simulink model "SUS_ST_GUI"  (R2014a)
settings: Solver=ode3  StartTime=0.0  StopTime=T  FixedStep=0.1  RelTol=1e-3
values from neighbouring files (symbols this model uses):
  CA = str2double(get(handles.CA,'string'))    [SUS_ST_0326.m]    (also in SUS_ST_GUI_0326.m)
  IN = str2double(get(handles.IN,'string'))    [SUS_ST_0326.m]    (also in SUS_ST_GUI_0326.m)
  LT = str2double(get(handles.LT,'string'))    [SUS_ST_GUI_0326.m]
  N = 1    [SUS_ST_0326.m]
  SR = str2double(get(handles.SR,'string'))    [SUS_ST_0326.m]    (also in SUS_ST_GUI_0326.m)
  ST = str2double(get(handles.ST,'string'))    [SUS_ST_GUI_0326.m]
  ST_S = str2double(get(handles.ST_S,'string'))    [SUS_ST_GUI_0326.m]
  T = 10    [SUS_ST_GUI_0326.m]
  T5 = str2double(get(handles.T5,'string'))    [SUS_ST_0326.m]    (also in SUS_ST_GUI_0326.m)
  T6 = str2double(get(handles.T6,'string'))    [SUS_ST_0326.m]    (also in SUS_ST_GUI_0326.m)
  X11 = (Z11-H/sind(CA)-b2_3)/k2_3    [SUS_ST_GUI_0326.m]
  X12 = (Z12-bb2_3)/k2_3    [SUS_ST_GUI_0326.m]
  X13 = X12-X12_3    [SUS_ST_GUI_0326.m]
  X14 = X9+X14_1    [SUS_ST_GUI_0326.m]
  X15 = X9+X15_1    [SUS_ST_GUI_0326.m]
  X16 = X9+X16_2    [SUS_ST_GUI_0326.m]
  X2 = -abs(Z3)*tand(CA)    [SUS_ST_GUI_0326.m]
  x2 = 0    [SUS_ST_GUI_0326.m]
  X3 = abs(Z2)*tand(CA)    [SUS_ST_GUI_0326.m]
  x3 = 0    [SUS_ST_GUI_0326.m]
  x4 = str2double(get(handles.x4,'string'))    [SUS_ST_0326.m]    (also in SUS_ST_GUI_0326.m)
  X5 = X4-a1*cosd(T5)    [SUS_ST_GUI_0326.m]
  x5 = 0    [SUS_ST_GUI_0326.m]
  X6 = X4+b1*cosd(T5)    [SUS_ST_GUI_0326.m]
  x6 = str2double(get(handles.x6,'string'))    [SUS_ST_0326.m]    (also in SUS_ST_GUI_0326.m)
  X7 = X1-a2*cosd(T6)    [SUS_ST_GUI_0326.m]
  x7 = x4-e7    [SUS_ST_GUI_0326.m]
  X8 = X1+b2*cosd(T6)    [SUS_ST_GUI_0326.m]
  x8 = x9-l8*sind(t8)    [SUS_ST_GUI_0326.m]
  X9 = str2double(get(handles.X9,'string'))    [SUS_ST_0326.m]    (also in SUS_ST_GUI_0326.m)
  x9 = str2double(get(handles.x9,'string'))    [SUS_ST_0326.m]    (also in SUS_ST_GUI_0326.m)
  XC1 = (X7+X2+X8)/3    [SUS_ST_GUI_0326.m]
  xc1 = (x3+x4+x5)/3    [SUS_ST_GUI_0326.m]
  XC2 = (X3+X2)/2    [SUS_ST_GUI_0326.m]
  XC3 = (X5+X3+X6)/3    [SUS_ST_GUI_0326.m]
  Y11 = M/2    [SUS_ST_GUI_0326.m]
  Y12 = (B11_12-BB2_3)/(K2_3-K11_12)    [SUS_ST_GUI_0326.m]
  Y13 = Y12-Y12_3    [SUS_ST_GUI_0326.m]
  Y14 = Y9+Y14_1    [SUS_ST_GUI_0326.m]
  Y15 = Y9+Y15_1    [SUS_ST_GUI_0326.m]
  Y16 = Y9+Y16_2    [SUS_ST_GUI_0326.m]
  Y2 = (Z2-Z9)/K2_3+Y9-SR    [SUS_ST_GUI_0326.m]
  y2 = Y1+l2*cosd(t2+T2)    [SUS_ST_GUI_0326.m]
  Y3 = (Z3-Z9)/K2_3+Y9-SR    [SUS_ST_GUI_0326.m]
  y3 = y4+l4*cosd(t4)    [SUS_ST_GUI_0326.m]
  y4 = str2double(get(handles.y4,'string'))    [SUS_ST_0326.m]    (also in SUS_ST_GUI_0326.m)
  Y5 = Y4    [SUS_ST_GUI_0326.m]
  y5 = y4+l5*cosd(t5)    [SUS_ST_GUI_0326.m]
  Y6 = Y4    [SUS_ST_GUI_0326.m]
  y6 = str2double(get(handles.y6,'string'))    [SUS_ST_0326.m]    (also in SUS_ST_GUI_0326.m)
  Y7 = Y1    [SUS_ST_GUI_0326.m]
  y7 = y4+l7*cosd(t7)    [SUS_ST_GUI_0326.m]
  Y8 = Y1    [SUS_ST_GUI_0326.m]
  y8 = y9+l8*cosd(t8)    [SUS_ST_GUI_0326.m]
  Y9 = str2double(get(handles.Y9,'string'))    [SUS_ST_0326.m]    (also in SUS_ST_GUI_0326.m)
  y9 = str2double(get(handles.y9,'string'))    [SUS_ST_0326.m]    (also in SUS_ST_GUI_0326.m)
  YC1 = (Y7+Y2+Y8)/3    [SUS_ST_GUI_0326.m]
  yc1 = (y3+y4+y5)/3    [SUS_ST_GUI_0326.m]
  YC2 = (Y3+Y2)/2    [SUS_ST_GUI_0326.m]
  YC3 = (Y5+Y3+Y6)/3    [SUS_ST_GUI_0326.m]
  Z11 = str2double(get(handles.Z11,'string'))    [SUS_ST_0326.m]    (also in SUS_ST_GUI_0326.m)
  Z12 = str2double(get(handles.Z12,'string'))    [SUS_ST_0326.m]    (also in SUS_ST_GUI_0326.m = K11_12*Y12+B11_12)
  Z13 = Z12-Z12_3    [SUS_ST_GUI_0326.m]
  Z14 = Z9+Z14_1    [SUS_ST_GUI_0326.m]
  Z15 = Z9+Z15_1    [SUS_ST_GUI_0326.m]
  Z16 = Z9+Z16_2    [SUS_ST_GUI_0326.m]
  Z2 = str2double(get(handles.Z2,'string'))    [SUS_ST_0326.m]    (also in SUS_ST_GUI_0326.m)
  z2 = Z1+l2*sind(t2+T2)    [SUS_ST_GUI_0326.m]
  Z3 = str2double(get(handles.Z3,'string'))    [SUS_ST_0326.m]    (also in SUS_ST_GUI_0326.m)
  z3 = z4+l4*sind(t4)    [SUS_ST_GUI_0326.m]
  z4 = str2double(get(handles.z4,'string'))    [SUS_ST_0326.m]    (also in SUS_ST_GUI_0326.m)
  Z5 = Z4-a1*sind(T5)    [SUS_ST_GUI_0326.m]
  z5 = z4+l5*sind(t5)    [SUS_ST_GUI_0326.m]
  Z6 = Z4+b1*sind(T5)    [SUS_ST_GUI_0326.m]
  z6 = str2double(get(handles.z6,'string'))    [SUS_ST_0326.m]    (also in SUS_ST_GUI_0326.m)
  Z7 = Z1-a2*sind(T6)    [SUS_ST_GUI_0326.m]
  z7 = z4+l7*sind(t7)    [SUS_ST_GUI_0326.m]
  Z8 = Z1+b2*sind(T6)    [SUS_ST_GUI_0326.m]
  z8 = z9    [SUS_ST_GUI_0326.m]
  Z9 = str2double(get(handles.Z9,'string'))    [SUS_ST_0326.m]    (also in SUS_ST_GUI_0326.m)
  z9 = str2double(get(handles.z9,'string'))    [SUS_ST_0326.m]    (also in SUS_ST_GUI_0326.m)
  ZC1 = (Z7+Z2+Z8)/3    [SUS_ST_GUI_0326.m]
  zc1 = (z3+z4+z5)/3    [SUS_ST_GUI_0326.m]
  ZC2 = (Z3+Z2)/2    [SUS_ST_GUI_0326.m]
  ZC3 = (Z5+Z3+Z6)/3    [SUS_ST_GUI_0326.m]
libraries: mblibv1 x79, simulink x3
(part 1 of 2)
settings Model: Creator=Administrator  LastModifiedBy=ZBingF
settings DebuggingCC: UnderspecifiedInitializationDetection=Classic  StateNameClashWarn=warning
settings SimMechanicsCC: VisDuringSimulation=on

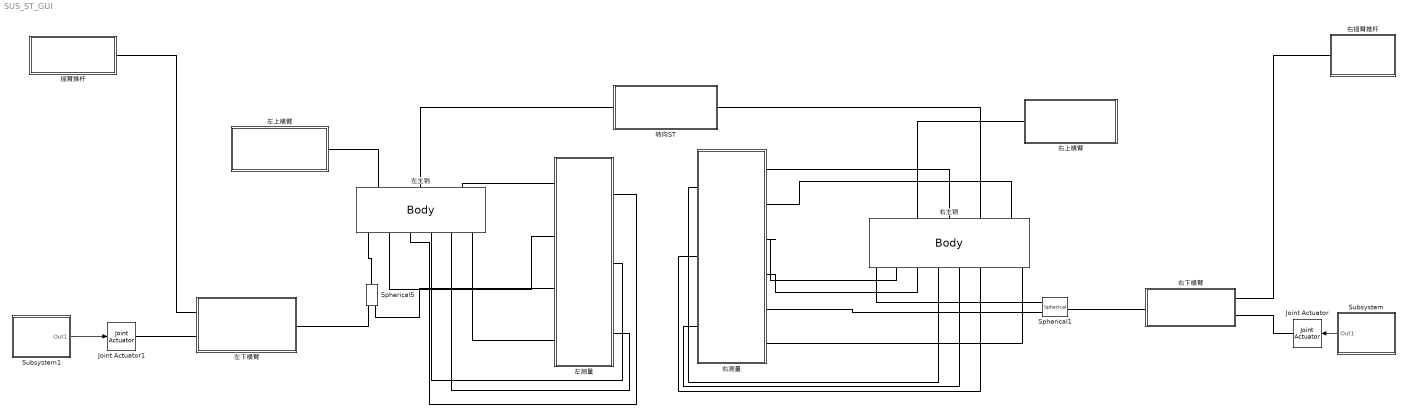
== system SUS_ST_GUI ==
  Joint Actuator : mblibv1/Sensors &  Actuators/Joint Actuator  UpdateFromCAD=off  PhysicalDomain=Mechanical  PortType=blob  ActuationStyle=Motion  AngleUnits=deg  ArcVelocityUnits=deg/s  ArcAccelerationUnits=deg/s^2  CoordPositionUnits=m  VelocityUnits=m/s  AccelerationUnits=m/s^2  ForceUnits=N  TorqueUnits=N*m  ActiveIO=on  Width=3  DialogClass=MechanicalActuatorBlock  Primitive=R1  ReferenceFrame=Absolute (World)
  Joint Actuator1 : mblibv1/Sensors &  Actuators/Joint Actuator  UpdateFromCAD=off  PhysicalDomain=Mechanical  PortType=blob  ActuationStyle=Motion  AngleUnits=deg  ArcVelocityUnits=deg/s  ArcAccelerationUnits=deg/s^2  CoordPositionUnits=m  VelocityUnits=m/s  AccelerationUnits=m/s^2  ForceUnits=N  TorqueUnits=N*m  ActiveIO=on  Width=3  DialogClass=MechanicalActuatorBlock  Primitive=R1  ReferenceFrame=Absolute (World)
  Spherical1 : mblibv1/Joints/Spherical  LConnTagsString=__newl0|SA1  RConnTagsString=__newr0  UpdateFromCAD=off  NumSAPorts=1  CutJoint=off  MarkAsCut=off  Primitives=spherical  PrimitiveProps=S$World$[0 0 0]$spherical  DialogClass=JointBlock  SAxis=[0 0 0]
  Spherical5 : mblibv1/Joints/Spherical  LConnTagsString=__newl0|SA1  RConnTagsString=__newr0  UpdateFromCAD=off  NumSAPorts=1  CutJoint=off  MarkAsCut=off  Primitives=spherical  PrimitiveProps=S$World$[0 0 0]$spherical  DialogClass=JointBlock  SAxis=[0 0 0]
  Subsystem : Subsystem
  Subsystem1 : Subsystem
  右上横臂 : Subsystem
  右下横臂 : Subsystem
  右主销 : mblibv1/Bodies/Body  LConnTagsString=CG|CS1|CS4|CS6|CS7  RConnTagsString=CS2|CS5|CS3|CS10|CS12|CS11|CS9|CS8  UpdateFromCAD=off  DialogClass=MechanicalBodyBlock  Mass=1  MassUnits=kg  InertiaUnits=kg*m^2  Inertia=eye(3)  Shape=Cylinder  ShapeDims=[1 1]  ShapeUnits=m  ShapeUse=false  Density=1  DensityUnits=kg/m^3  DensityUse=false  GraphicsMode=MACHINE_DEFAULT  BodyColorSelMode=MACHINE_DEFAULT  BodyColor=[1 0 0]  AttachedToCS=CG  CG=Left$CG$[XC2 YC2 ZC2]$WORLD$WORLD$mm$[0 0 0]$Euler X-Y-Z$deg$WORLD$true$none  WorkingFrames=Left$CS1$[X3 Y3 Z3]$World$World$mm$[0 0 0]$Euler X-Y-Z$deg$WORLD$true$none#Left$CS4$[X3 Y3 Z3]$World$World$mm$[0 0 0]$Euler X-Y-Z$deg$WORLD$true$none#Right$CS2$[X2 Y2 Z2]$World$World$mm$[IN CA 0]$Euler X-Y-Z$deg$WORLD$true$none#Right$CS5$[X2 Y2 Z2]$World$World$mm$[0 0 0]$Euler X-Y-Z$deg$WORLD$true$none#Right$CS3$[X9 Y9 Z9]$World$World$mm$[0 0 0]$Euler X-Y-Z$deg$WORLD$true$none#Right$CS10$[X14 Y14 Z14]$World$World$mm$[0 0 0]$Euler X-Y-Z$deg$WORLD$true$none#Right$CS12$[X16 Y16 Z16]$World$World$mm$[0 0 0]$Euler X-Y-Z$deg$WORLD$true$none#Right$CS11$[X15 Y15 Z15]$World$World$mm$[0 0 0]$Euler X-Y-Z$deg$WORLD$true$none#Right$CS9$[X9 Y9-SR Z9]$World$World$mm$[IN CA 0]$Euler X-Y-Z$deg$WORLD$true$none#Left$CS6$[X12 Y12 Z12]$World$World$mm$[0 0 0]$Euler X-Y-Z$deg$WORLD$true$none#Left$CS7$[X12 Y12 Z12]$World$World$mm$[0 0 0]$Euler X-Y-Z$deg$WORLD$true$none#Right$CS8$[X13 Y13 Z13]$World$World$mm$[0 0 0]$Euler X-Y-Z$deg$WORLD$true$none  CGPos=[XC2 YC2 ZC2]  CGRot=[0 0 0]  CS0Pos=[]  CS0Rot=[]  CS1Pos=[X3 Y3 Z3]  CS1Rot=[0 0 0]  CS2Pos=[X2 Y2 Z2]  CS2Rot=[IN CA 0]  CS3Pos=[X9 Y9 Z9]  CS3Rot=[0 0 0]  CS4Pos=[X3 Y3 Z3]  CS4Rot=[0 0 0]  CS5Pos=[X2 Y2 Z2]  CS5Rot=[0 0 0]  CS6Pos=[X12 Y12 Z12]  CS6Rot=[0 0 0]  CS7Pos=[X12 Y12 Z12]  CS7Rot=[0 0 0]  CS8Pos=[X13 Y13 Z13]  CS8Rot=[0 0 0]  CS9Pos=[X9 Y9-SR Z9]  CS9Rot=[IN CA 0]  CS10Pos=[X14 Y14 Z14]  CS10Rot=[0 0 0]  CS11Pos=[X15 Y15 Z15]  CS11Rot=[0 0 0]  CS12Pos=[X16 Y16 Z16]  CS12Rot=[0 0 0]  CS13Pos=[]  CS13Rot=[]  CS14Pos=[]  CS14Rot=[]  CS15Pos=[]  CS15Rot=[]  CS16Pos=[]  CS16Rot=[]  CS17Pos=[]  CS17Rot=[]  CS18Pos=[]  CS18Rot=[]  CS19Pos=[]  CS19Rot=[]  CS20Pos=[]  CS20Rot=[]
  右摇臂推杆 : Subsystem
  右测量 : Subsystem
  左上横臂 : Subsystem
  左下横臂 : Subsystem
  左主销 : mblibv1/Bodies/Body  LConnTagsString=CS1|CS6|CS7  RConnTagsString=CS2|CS3|CS9|CS10|CS11|CS8  UpdateFromCAD=off  DialogClass=MechanicalBodyBlock  Mass=1  MassUnits=kg  InertiaUnits=kg*m^2  Inertia=eye(3)  Shape=Cylinder  ShapeDims=[1 1]  ShapeUnits=m  ShapeUse=false  Density=1  DensityUnits=kg/m^3  DensityUse=false  GraphicsMode=MACHINE_DEFAULT  BodyColorSelMode=MACHINE_DEFAULT  BodyColor=[1 0 0]  AttachedToCS=CG  CG=Left$CG$[XC2 -YC2 ZC2]$WORLD$WORLD$mm$[0 0 0]$Euler X-Y-Z$deg$WORLD$false$none  WorkingFrames=Left$CS1$[X3 -Y3 Z3]$World$World$mm$[0 0 0]$Euler X-Y-Z$deg$WORLD$true$none#Left$CS4$[X3 -Y3 Z3]$World$World$mm$[0 0 0]$Euler X-Y-Z$deg$WORLD$false$none#Right$CS2$[X2 -Y2 Z2]$World$World$mm$[-IN CA 0]$Euler X-Y-Z$deg$WORLD$true$none#Right$CS5$[X2 -Y2 Z2]$World$World$mm$[0 0 0]$Euler X-Y-Z$deg$WORLD$false$none#Right$CS3$[X9 -Y9 Z9]$World$World$mm$[0 0 0]$Euler X-Y-Z$deg$WORLD$true$none#Right$CS9$[X14 -Y14 Z14]$World$World$mm$[0 0 0]$Euler X-Y-Z$deg$WORLD$true$none#Right$CS10$[X15 -Y15 Z15]$World$World$mm$[0 0 0]$Euler X-Y-Z$deg$WORLD$true$none#Right$CS11$[X16 -Y16 Z16]$World$World$mm$[0 0 0]$Euler X-Y-Z$deg$WORLD$true$none#Right$CS8$[X13 -Y13 Z13]$World$World$mm$[0 0 0]$Euler X-Y-Z$deg$WORLD$true$none#Left$CS6$[X12 -Y12 Z12]$World$World$mm$[0 0 0]$Euler X-Y-Z$deg$WORLD$true$none#Left$CS7$[X12 -Y12 Z12]$World$World$mm$[0 0 0]$Euler X-Y-Z$deg$WORLD$true$none  CGPos=[XC2 -YC2 ZC2]  CGRot=[0 0 0]  CS0Pos=[]  CS0Rot=[]  CS1Pos=[X3 -Y3 Z3]  CS1Rot=[0 0 0]  CS2Pos=[X2 -Y2 Z2]  CS2Rot=[-IN CA 0]  CS3Pos=[X9 -Y9 Z9]  CS3Rot=[0 0 0]  CS4Pos=[X3 -Y3 Z3]  CS4Rot=[0 0 0]  CS5Pos=[X2 -Y2 Z2]  CS5Rot=[0 0 0]  CS6Pos=[X12 -Y12 Z12]  CS6Rot=[0 0 0]  CS7Pos=[X12 -Y12 Z12]  CS7Rot=[0 0 0]  CS8Pos=[X13 -Y13 Z13]  CS8Rot=[0 0 0]  CS9Pos=[X14 -Y14 Z14]  CS9Rot=[0 0 0]  CS10Pos=[X15 -Y15 Z15]  CS10Rot=[0 0 0]  CS11Pos=[X16 -Y16 Z16]  CS11Rot=[0 0 0]  CS12Pos=[]  CS12Rot=[]  CS13Pos=[]  CS13Rot=[]  CS14Pos=[]  CS14Rot=[]  CS15Pos=[]  CS15Rot=[]  CS16Pos=[]  CS16Rot=[]  CS17Pos=[]  CS17Rot=[]  CS18Pos=[]  CS18Rot=[]  CS19Pos=[]  CS19Rot=[]  CS20Pos=[]  CS20Rot=[]
  左测量 : Subsystem
  摇臂推杆 : Subsystem
  转向ST : Subsystem
  wires:
  Subsystem/1(Out1) -> Joint Actuator/1
  Subsystem1/1(Out1) -> Joint Actuator1/1
  connections:
  右主销/RConn1 -- Spherical1/LConn1
  Spherical5/RConn1 -- 左主销/RConn1
  左主销/LConn2 -- 转向ST/LConn1
  右主销/LConn4 -- 转向ST/RConn1
  左上横臂/LConn1 -- 左主销/LConn1
  左下横臂/LConn1 -- 摇臂推杆/RConn1
  左下横臂/RConn1 -- Spherical5/LConn1
  Joint Actuator1/RConn1 -- 左下横臂/LConn2
  右主销/LConn2 -- 右上横臂/LConn1
  右摇臂推杆/RConn1 -- 右下横臂/LConn1
  右下横臂/RConn1 -- Spherical1/RConn1
  Joint Actuator/RConn1 -- 右下横臂/LConn2
  右测量/RConn1 -- 右主销/LConn3
  右测量/RConn2 -- 右主销/LConn5
  右测量/RConn3 -- 右主销/RConn2
  右测量/RConn4 -- 右主销/RConn3
  右测量/RConn5 -- Spherical1/LConn2
  左测量/LConn1 -- 左主销/LConn3
  左主销/RConn2 -- 左测量/LConn2
  左测量/LConn3 -- Spherical5/LConn2
  左测量/LConn4 -- 左主销/RConn6
  右测量/RConn6 -- 右主销/RConn8
  右测量/LConn1 -- 右主销/RConn4
  右测量/LConn2 -- 右主销/RConn6
  左测量/RConn1 -- 左主销/RConn3
  左测量/RConn2 -- 左主销/RConn4
  右测量/LConn3 -- 右主销/RConn5
  左主销/RConn5 -- 左测量/RConn3

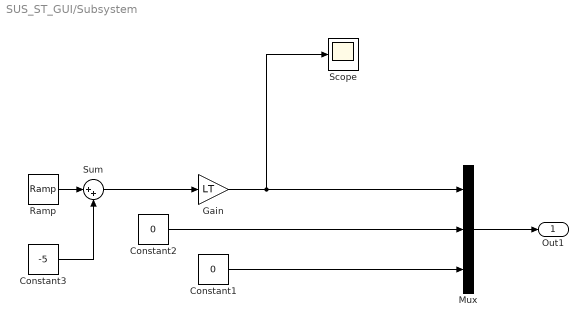
== system SUS_ST_GUI/Subsystem ==
  Constant1 : Constant  Value=0
  Constant2 : Constant  Value=0
  Constant3 : Constant  Value=-5
  Gain : Gain  Gain=LT
  Mux : Mux  Inputs=3
  Ramp : simulink/Sources/Ramp  slope=1  start=0  X0=0
  Scope : Scope
      settings: SaveName=ScopeData3
  Sum : Sum  Inputs=|++
  Out1 : Outport
  wires:
  Mux/1 -> Out1/1
  Gain/1 -> Scope/1, Mux/1
  Constant1/1 -> Mux/3
  Constant2/1 -> Mux/2
  Ramp/1 -> Sum/1
  Constant3/1 -> Sum/2
  Sum/1 -> Gain/1

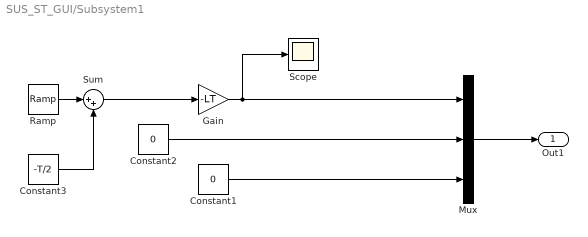
== system SUS_ST_GUI/Subsystem1 ==
  Constant1 : Constant  Value=0
  Constant2 : Constant  Value=0
  Constant3 : Constant  Value=-T/2
  Gain : Gain  Gain=-LT
  Mux : Mux  Inputs=3
  Ramp : simulink/Sources/Ramp  slope=1  start=0  X0=0
  Scope : Scope
      settings: SaveName=ScopeData2
  Sum : Sum  Inputs=|++
  Out1 : Outport
  wires:
  Mux/1 -> Out1/1
  Gain/1 -> Scope/1, Mux/1
  Constant1/1 -> Mux/3
  Constant2/1 -> Mux/2
  Ramp/1 -> Sum/1
  Constant3/1 -> Sum/2
  Sum/1 -> Gain/1

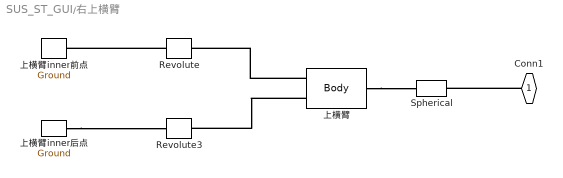
== system SUS_ST_GUI/右上横臂 ==
  Revolute : mblibv1/Joints/Revolute  LConnTagsString=__newl0  RConnTagsString=__newr0  UpdateFromCAD=off  NumSAPorts=0  CutJoint=off  MarkAsCut=off  Primitives=prismatic  PrimitiveProps=R1$World$[cosd(T5) 0 sind(T5)]$revolute  DialogClass=JointBlock  R1Axis=[cosd(T5) 0 sind(T5)]
  Revolute3 : mblibv1/Joints/Revolute  LConnTagsString=__newl0  RConnTagsString=__newr0  UpdateFromCAD=off  NumSAPorts=0  CutJoint=off  MarkAsCut=off  Primitives=prismatic  PrimitiveProps=R1$World$[cosd(T5) 0 sind(T5)]$revolute  DialogClass=JointBlock  R1Axis=[cosd(T5) 0 sind(T5)]
  Spherical : mblibv1/Joints/Spherical  LConnTagsString=__newl0  RConnTagsString=__newr0  UpdateFromCAD=off  NumSAPorts=0  CutJoint=off  MarkAsCut=off  Primitives=spherical  PrimitiveProps=S$World$[0 0 0]$spherical  DialogClass=JointBlock  SAxis=[0 0 0]
  上横臂 : mblibv1/Bodies/Body  LConnTagsString=CS1|CS3  RConnTagsString=CS2  UpdateFromCAD=off  DialogClass=MechanicalBodyBlock  Mass=1  MassUnits=kg  InertiaUnits=kg*m^2  Inertia=eye(3)  Shape=Cylinder  ShapeDims=[1 1]  ShapeUnits=m  ShapeUse=false  Density=1  DensityUnits=kg/m^3  DensityUse=false  GraphicsMode=MACHINE_DEFAULT  BodyColorSelMode=MACHINE_DEFAULT  BodyColor=[1 0 0]  AttachedToCS=CG  CG=Left$CG$[XC3 YC3 ZC3]$WORLD$WORLD$mm$[0 0 0]$Euler X-Y-Z$deg$WORLD$false$none  WorkingFrames=Left$CS1$[X5 Y5 Z5]$World$World$mm$[0 0 0]$Euler X-Y-Z$deg$WORLD$true$none#Right$CS2$[X3 Y3 Z3]$World$World$mm$[0 0 0]$Euler X-Y-Z$deg$WORLD$true$none#Left$CS3$[X6 Y6 Z6]$World$World$mm$[0 0 0]$Euler X-Y-Z$deg$WORLD$true$none  CGPos=[XC3 YC3 ZC3]  CGRot=[0 0 0]  CS0Pos=[]  CS0Rot=[]  CS1Pos=[X5 Y5 Z5]  CS1Rot=[0 0 0]  CS2Pos=[X3 Y3 Z3]  CS2Rot=[0 0 0]  CS3Pos=[X6 Y6 Z6]  CS3Rot=[0 0 0]  CS4Pos=[]  CS4Rot=[]  CS5Pos=[]  CS5Rot=[]  CS6Pos=[]  CS6Rot=[]  CS7Pos=[]  CS7Rot=[]  CS8Pos=[]  CS8Rot=[]  CS9Pos=[]  CS9Rot=[]  CS10Pos=[]  CS10Rot=[]  CS11Pos=[]  CS11Rot=[]  CS12Pos=[]  CS12Rot=[]  CS13Pos=[]  CS13Rot=[]  CS14Pos=[]  CS14Rot=[]  CS15Pos=[]  CS15Rot=[]  CS16Pos=[]  CS16Rot=[]  CS17Pos=[]  CS17Rot=[]  CS18Pos=[]  CS18Rot=[]  CS19Pos=[]  CS19Rot=[]  CS20Pos=[]  CS20Rot=[]
  上横臂inner前点 : mblibv1/Bodies/Ground  UpdateFromCAD=off  LeftPortType=env  RightPortType=workingframe  PhysicalDomain=Mechanical  DialogClass=GroundBlock  CoordPosition=[X5 Y5 Z5]  CoordPositionUnits=mm  StateVectorMgrId=-1  MachineId=[0 0]  ShowEnvPort=off  ParameterChecksum=[0 0 0 0]  TopologyChecksum=[0 0 0 0]
  上横臂inner后点 : mblibv1/Bodies/Ground  UpdateFromCAD=off  LeftPortType=env  RightPortType=workingframe  PhysicalDomain=Mechanical  DialogClass=GroundBlock  CoordPosition=[X6 Y6 Z6]  CoordPositionUnits=mm  StateVectorMgrId=-1  MachineId=[0 0]  ShowEnvPort=off  ParameterChecksum=[0 0 0 0]  TopologyChecksum=[0 0 0 0]
  Conn1 : PMIOPort  Port=1  Side=Left
  connections:
  Revolute/LConn1 -- 上横臂inner前点/RConn1
  上横臂/RConn1 -- Spherical/LConn1
  Conn1/RConn1 -- Spherical/RConn1
  上横臂/LConn2 -- Revolute3/RConn1
  上横臂inner后点/RConn1 -- Revolute3/LConn1
  上横臂/LConn1 -- Revolute/RConn1

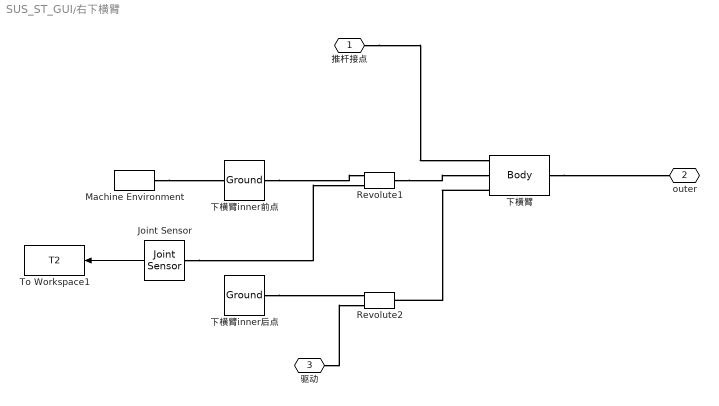
== system SUS_ST_GUI/右下横臂 ==
  Joint Sensor : mblibv1/Sensors &  Actuators/Joint Sensor  UpdateFromCAD=off  PhysicalDomain=Mechanical  PortType=blob  Muxed=on  Pose=off  Angle=on  AngleUnits=deg  ArcVelocity=off  ArcVelocityUnits=deg/s  ArcAcceleration=off  ArcAccelerationUnits=deg/s^2  CoordPosition=on  CoordPositionUnits=m  Velocity=off  VelocityUnits=m/s  Acceleration=off  AccelerationUnits=m/s^2  Quaternion=on  QuaternionDT=off  QuaternionDDT=off  QuaternionUnits=off  OutputVector=[1]  ActiveIO=on  Width=1  DialogClass=MechanicalSensorBlock  Primitive=R1  Force=off  ForceUnits=N  Torque=off  TorqueUnits=N-m  ReferenceFrame=Absolute (World)  ReactionSensedSide=Base  ReactionReferenceFrame=Absolute (World)  ReactionForce=off  ReactionForceUnits=N  ReactionMoment=off  ReactionMomentUnits=N-m
  Machine Environment : mblibv1/Bodies/Machine Environment  PortType=env  PhysicalDomain=Mechanical  DialogTemplateClass=MECH.MachineEnvironment  SyncWhenCopied=off  Gravity=[0 0 -9.81]  GravityUnits=m/s^2  GravityAsSignal=off  Dimensionality=Auto-detect  AnalysisType=Forward dynamics  LinearAssemblyTolerance=1e-3  LinearAssemblyToleranceUnits=m  AngularAssemblyTolerance=1e-3  AngularAssemblyToleranceUnits=rad  ConstraintSolverType=Stabilizing  ConstraintRelTolerance=1e-4  ConstraintAbsTolerance=1e-4  UseRobustSingularityHandling=off  RedundancyAnalysisToleranceType=Automatically select tolerance  RedundancyAnalysisTolerance=1e-14  StatePerturbationType=Fixed  PerturbationSize=1e-5  VisualizeMachine=on  BodyVisualizationType=Use model default body geometries  BodyColorSelMode=Use model default  DefaultBodyColor=[1 0 0]
  Revolute1 : mblibv1/Joints/Revolute  LConnTagsString=__newl0|SA1  RConnTagsString=__newr0  UpdateFromCAD=off  NumSAPorts=1  CutJoint=off  MarkAsCut=off  Primitives=prismatic  PrimitiveProps=R1$World$[cosd(T6) 0 sind(T6)]$revolute  DialogClass=JointBlock  R1Axis=[cosd(T6) 0 sind(T6)]
  Revolute2 : mblibv1/Joints/Revolute  LConnTagsString=__newl0|SA1  RConnTagsString=__newr0  UpdateFromCAD=off  NumSAPorts=1  CutJoint=off  MarkAsCut=off  Primitives=prismatic  PrimitiveProps=R1$World$[cosd(T6) 0 sind(T6)]$revolute  DialogClass=JointBlock  R1Axis=[cosd(T6) 0 sind(T6)]
  To Workspace1 : ToWorkspace  VariableName=T2  SampleTime=-1
      settings: RequirementInfo={} %GIDa_a5ba983f_6511_497d_a9a3_d28980eaffcb
  下横臂 : mblibv1/Bodies/Body  LConnTagsString=CS3|CS1|CS4  RConnTagsString=CS2  UpdateFromCAD=off  DialogClass=MechanicalBodyBlock  Mass=1  MassUnits=kg  InertiaUnits=kg*m^2  Inertia=eye(3)  Shape=Cylinder  ShapeDims=[1 1]  ShapeUnits=m  ShapeUse=false  Density=1  DensityUnits=kg/m^3  DensityUse=false  GraphicsMode=MACHINE_DEFAULT  BodyColorSelMode=MACHINE_DEFAULT  BodyColor=[1 0 0]  AttachedToCS=CG  CG=Left$CG$[XC1 YC1 ZC1]$WORLD$WORLD$mm$[0 0 0]$Euler X-Y-Z$deg$WORLD$false$none  WorkingFrames=Left$CS3$[x2 y2 z2]$WORLD$WORLD$mm$[0 0 0]$Euler X-Y-Z$deg$WORLD$true$none#Left$CS1$[X7 Y7 Z7]$World$World$mm$[0 0 0]$Euler X-Y-Z$deg$WORLD$true$none#Right$CS2$[X2 Y2 Z2]$World$World$mm$[IN CA 0]$Euler X-Y-Z$deg$WORLD$true$none#Left$CS4$[X8 Y8 Z8]$World$World$mm$[0 0 0]$Euler X-Y-Z$deg$WORLD$true$none  CGPos=[XC1 YC1 ZC1]  CGRot=[0 0 0]  CS0Pos=[]  CS0Rot=[]  CS1Pos=[X7 Y7 Z7]  CS1Rot=[0 0 0]  CS2Pos=[X2 Y2 Z2]  CS2Rot=[IN CA 0]  CS3Pos=[x2 y2 z2]  CS3Rot=[0 0 0]  CS4Pos=[X8 Y8 Z8]  CS4Rot=[0 0 0]  CS5Pos=[]  CS5Rot=[]  CS6Pos=[]  CS6Rot=[]  CS7Pos=[]  CS7Rot=[]  CS8Pos=[]  CS8Rot=[]  CS9Pos=[]  CS9Rot=[]  CS10Pos=[]  CS10Rot=[]  CS11Pos=[]  CS11Rot=[]  CS12Pos=[]  CS12Rot=[]  CS13Pos=[]  CS13Rot=[]  CS14Pos=[]  CS14Rot=[]  CS15Pos=[]  CS15Rot=[]  CS16Pos=[]  CS16Rot=[]  CS17Pos=[]  CS17Rot=[]  CS18Pos=[]  CS18Rot=[]  CS19Pos=[]  CS19Rot=[]  CS20Pos=[]  CS20Rot=[]
  下横臂inner前点 : mblibv1/Bodies/Ground  UpdateFromCAD=off  LeftPortType=env  RightPortType=workingframe  PhysicalDomain=Mechanical  DialogClass=GroundBlock  CoordPosition=[X7 Y7 Z7]  CoordPositionUnits=mm  StateVectorMgrId=0  MachineId=[1 0]  ShowEnvPort=on  ParameterChecksum=[3479177666, 2216579070, 775339487, 3024718770]  TopologyChecksum=[3339210118, 1670250069, 763971536, 2455140559]
  下横臂inner后点 : mblibv1/Bodies/Ground  UpdateFromCAD=off  LeftPortType=env  RightPortType=workingframe  PhysicalDomain=Mechanical  DialogClass=GroundBlock  CoordPosition=[X8 Y8 Z8]  CoordPositionUnits=mm  StateVectorMgrId=-1  MachineId=[0 0]  ShowEnvPort=off  ParameterChecksum=[0 0 0 0]  TopologyChecksum=[0 0 0 0]
  推杆接点 : PMIOPort  Port=1  Side=Left
  outer : PMIOPort  Port=2  Side=Right
  驱动 : PMIOPort  Port=3  Side=Left
  wires:
  Joint Sensor/1 -> To Workspace1/1
  connections:
  下横臂/RConn1 -- outer/RConn1
  Revolute1/RConn1 -- 下横臂/LConn2
  下横臂inner后点/RConn1 -- Revolute2/LConn1
  Machine Environment/RConn1 -- 下横臂inner前点/LConn1
  下横臂/LConn3 -- Revolute2/RConn1
  下横臂inner前点/RConn1 -- Revolute1/LConn1
  驱动/RConn1 -- Revolute2/LConn2
  推杆接点/RConn1 -- 下横臂/LConn1
  Joint Sensor/LConn1 -- Revolute1/LConn2

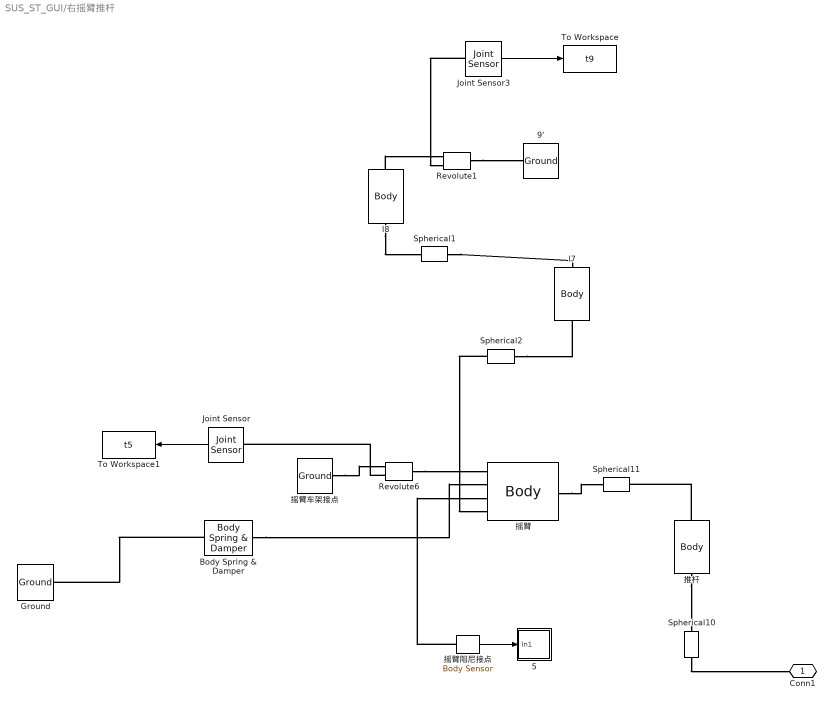
== system SUS_ST_GUI/右摇臂推杆 ==
  5 : Subsystem
  9‘ : mblibv1/Bodies/Ground  UpdateFromCAD=off  LeftPortType=env  RightPortType=workingframe  PhysicalDomain=Mechanical  DialogClass=GroundBlock  CoordPosition=[x9,y9,z9]  CoordPositionUnits=mm  StateVectorMgrId=-1  MachineId=[0 0]  ShowEnvPort=off  ParameterChecksum=[0 0 0 0]  TopologyChecksum=[0 0 0 0]
  Body Spring & Damper : mblibv1/Force  Elements/Body Spring & Damper  UpdateFromCAD=off  DialogClass=BodySpringDamper  Spring_k=0  Damper_b=0  Offset_x0=0  PositionUnits=m  VelocityUnits=m/s  ForceUnits=N
  Ground : mblibv1/Bodies/Ground  UpdateFromCAD=off  LeftPortType=env  RightPortType=workingframe  PhysicalDomain=Mechanical  DialogClass=GroundBlock  CoordPosition=[x6 y6 z6]  CoordPositionUnits=mm  StateVectorMgrId=-1  MachineId=[0 0]  ShowEnvPort=off  ParameterChecksum=[0 0 0 0]  TopologyChecksum=[0 0 0 0]
  Joint Sensor : mblibv1/Sensors &  Actuators/Joint Sensor  UpdateFromCAD=off  PhysicalDomain=Mechanical  PortType=blob  Muxed=on  Pose=off  Angle=on  AngleUnits=deg  ArcVelocity=off  ArcVelocityUnits=deg/s  ArcAcceleration=off  ArcAccelerationUnits=deg/s^2  CoordPosition=on  CoordPositionUnits=m  Velocity=off  VelocityUnits=m/s  Acceleration=off  AccelerationUnits=m/s^2  Quaternion=on  QuaternionDT=off  QuaternionDDT=off  QuaternionUnits=off  OutputVector=[1]  ActiveIO=on  Width=1  DialogClass=MechanicalSensorBlock  Primitive=R1  Force=off  ForceUnits=N  Torque=off  TorqueUnits=N-m  ReferenceFrame=Absolute (World)  ReactionSensedSide=Base  ReactionReferenceFrame=Absolute (World)  ReactionForce=off  ReactionForceUnits=N  ReactionMoment=off  ReactionMomentUnits=N-m
  Joint Sensor3 : mblibv1/Sensors &  Actuators/Joint Sensor  RequirementInfo={} %GIDa_7025f6a4_6e00_4f62_b684_7bfb1a25e7a0  UpdateFromCAD=off  PhysicalDomain=Mechanical  PortType=blob  Muxed=on  Pose=off  Angle=on  AngleUnits=deg  ArcVelocity=off  ArcVelocityUnits=deg/s  ArcAcceleration=off  ArcAccelerationUnits=deg/s^2  CoordPosition=on  CoordPositionUnits=m  Velocity=off  VelocityUnits=m/s  Acceleration=off  AccelerationUnits=m/s^2  Quaternion=on  QuaternionDT=off  QuaternionDDT=off  QuaternionUnits=off  OutputVector=[1]  ActiveIO=on  Width=1  DialogClass=MechanicalSensorBlock  Primitive=R1  Force=off  ForceUnits=N  Torque=off  TorqueUnits=N*m  ReferenceFrame=Absolute (World)  ReactionSensedSide=Follower  ReactionReferenceFrame=Local (Body CS)  ReactionForce=off  ReactionForceUnits=N  ReactionMoment=off  ReactionMomentUnits=N*m
  Revolute1 : mblibv1/Joints/Revolute  LConnTagsString=__newl0|SA1  RConnTagsString=__newr0  UpdateFromCAD=off  NumSAPorts=1  CutJoint=off  MarkAsCut=off  Primitives=prismatic  PrimitiveProps=R1$World$[0 0 1]$revolute  DialogClass=JointBlock  R1Axis=[0 0 1]
  Revolute6 : mblibv1/Joints/Revolute  LConnTagsString=__newl0|SA1  RConnTagsString=__newr0  UpdateFromCAD=off  NumSAPorts=1  CutJoint=off  MarkAsCut=off  Primitives=prismatic  PrimitiveProps=R1$World$[1 0 0]$revolute  DialogClass=JointBlock  R1Axis=[1 0 0]
  Spherical{1..2,10..11} (4 alike) : mblibv1/Joints/Spherical  LConnTagsString=__newl0  RConnTagsString=__newr0  UpdateFromCAD=off  NumSAPorts=0  CutJoint=off  MarkAsCut=off  Primitives=spherical  PrimitiveProps=S$WORLD$[0 0 0]$spherical  DialogClass=JointBlock  SAxis=[0 0 0]
  To Workspace : ToWorkspace  VariableName=t9  SampleTime=-1
      settings: RequirementInfo={} %GIDa_ce77e2e2_e9bc_4260_90a1_1d22490a9ae3
  To Workspace1 : ToWorkspace  VariableName=t5  SampleTime=-1
      settings: RequirementInfo={} %GIDa_33bb5ac6_5f33_4822_af4d_f7cf8030d507
  l7 : mblibv1/Bodies/Body  LConnTagsString=CS1  RConnTagsString=CS2  UpdateFromCAD=off  DialogClass=MechanicalBodyBlock  Mass=1  MassUnits=kg  InertiaUnits=kg*m^2  Inertia=eye(3)  Shape=Cylinder  ShapeDims=[1 1]  ShapeUnits=m  ShapeUse=false  Density=1  DensityUnits=kg/m^3  DensityUse=false  GraphicsMode=MACHINE_DEFAULT  BodyColorSelMode=MACHINE_DEFAULT  BodyColor=[1 0 0]  AttachedToCS=CG  CG=Left$CG$[(x8+x7)/2 (y7+y8)/2 (z8+z7)/2]$WORLD$WORLD$mm$[0 0 0]$Euler X-Y-Z$deg$WORLD$false$none  WorkingFrames=Left$CS1$[x8,y8,z8]$World$World$mm$[0 0 0]$Euler X-Y-Z$deg$WORLD$true$none#Right$CS2$[x7 y7 z7]$World$World$mm$[0 0 0]$Euler X-Y-Z$deg$WORLD$true$none  CGPos=[(x8+x7)/2 (y7+y8)/2 (z8+z7)/2]  CGRot=[0 0 0]  CS0Pos=[]  CS0Rot=[]  CS1Pos=[x8,y8,z8]  CS1Rot=[0 0 0]  CS2Pos=[x7 y7 z7]  CS2Rot=[0 0 0]  CS3Pos=[]  CS3Rot=[]  CS4Pos=[]  CS4Rot=[]  CS5Pos=[]  CS5Rot=[]  CS6Pos=[]  CS6Rot=[]  CS7Pos=[]  CS7Rot=[]  CS8Pos=[]  CS8Rot=[]  CS9Pos=[]  CS9Rot=[]  CS10Pos=[]  CS10Rot=[]  CS11Pos=[]  CS11Rot=[]  CS12Pos=[]  CS12Rot=[]  CS13Pos=[]  CS13Rot=[]  CS14Pos=[]  CS14Rot=[]  CS15Pos=[]  CS15Rot=[]  CS16Pos=[]  CS16Rot=[]  CS17Pos=[]  CS17Rot=[]  CS18Pos=[]  CS18Rot=[]  CS19Pos=[]  CS19Rot=[]  CS20Pos=[]  CS20Rot=[]
  "l8 " : mblibv1/Bodies/Body  LConnTagsString=CS1  RConnTagsString=CS2  UpdateFromCAD=off  DialogClass=MechanicalBodyBlock  Mass=1  MassUnits=kg  InertiaUnits=kg*m^2  Inertia=eye(3)  Shape=Cylinder  ShapeDims=[1 1]  ShapeUnits=m  ShapeUse=false  Density=1  DensityUnits=kg/m^3  DensityUse=false  GraphicsMode=MACHINE_DEFAULT  BodyColorSelMode=MACHINE_DEFAULT  BodyColor=[1 0 0]  AttachedToCS=CG  CG=Left$CG$[(x8+x9)/2 (y9+y8)/2 (z8+z9)/2]$WORLD$WORLD$mm$[0 0 0]$Euler X-Y-Z$deg$WORLD$false$none  WorkingFrames=Left$CS1$[x8,y8,z8]$World$World$mm$[0 0 0]$Euler X-Y-Z$deg$WORLD$true$none#Right$CS2$[x9,y9,z9]$World$World$mm$[0 0 0]$Euler X-Y-Z$deg$WORLD$true$none  CGPos=[(x8+x9)/2 (y9+y8)/2 (z8+z9)/2]  CGRot=[0 0 0]  CS0Pos=[]  CS0Rot=[]  CS1Pos=[x8,y8,z8]  CS1Rot=[0 0 0]  CS2Pos=[x9,y9,z9]  CS2Rot=[0 0 0]  CS3Pos=[]  CS3Rot=[]  CS4Pos=[]  CS4Rot=[]  CS5Pos=[]  CS5Rot=[]  CS6Pos=[]  CS6Rot=[]  CS7Pos=[]  CS7Rot=[]  CS8Pos=[]  CS8Rot=[]  CS9Pos=[]  CS9Rot=[]  CS10Pos=[]  CS10Rot=[]  CS11Pos=[]  CS11Rot=[]  CS12Pos=[]  CS12Rot=[]  CS13Pos=[]  CS13Rot=[]  CS14Pos=[]  CS14Rot=[]  CS15Pos=[]  CS15Rot=[]  CS16Pos=[]  CS16Rot=[]  CS17Pos=[]  CS17Rot=[]  CS18Pos=[]  CS18Rot=[]  CS19Pos=[]  CS19Rot=[]  CS20Pos=[]  CS20Rot=[]
  推杆 : mblibv1/Bodies/Body  LConnTagsString=CS1  RConnTagsString=CS2  UpdateFromCAD=off  DialogClass=MechanicalBodyBlock  Mass=1  MassUnits=kg  InertiaUnits=kg*m^2  Inertia=eye(3)  Shape=Cylinder  ShapeDims=[1 1]  ShapeUnits=m  ShapeUse=false  Density=1  DensityUnits=kg/m^3  DensityUse=false  GraphicsMode=MACHINE_DEFAULT  BodyColorSelMode=MACHINE_DEFAULT  BodyColor=[1 0 0]  AttachedToCS=CG  CG=Left$CG$[(x2+x3)/2 (y3+y2)/2 (z2+z3)/2]$WORLD$WORLD$mm$[0 0 0]$Euler X-Y-Z$deg$WORLD$false$none  WorkingFrames=Left$CS1$[x2 y2 z2]$World$World$mm$[0 0 0]$Euler X-Y-Z$deg$WORLD$true$none#Right$CS2$[x3 y3 z3]$World$World$mm$[0 0 0]$Euler X-Y-Z$deg$WORLD$true$none  CGPos=[(x2+x3)/2 (y3+y2)/2 (z2+z3)/2]  CGRot=[0 0 0]  CS0Pos=[]  CS0Rot=[]  CS1Pos=[x2 y2 z2]  CS1Rot=[0 0 0]  CS2Pos=[x3 y3 z3]  CS2Rot=[0 0 0]  CS3Pos=[]  CS3Rot=[]  CS4Pos=[]  CS4Rot=[]  CS5Pos=[]  CS5Rot=[]  CS6Pos=[]  CS6Rot=[]  CS7Pos=[]  CS7Rot=[]  CS8Pos=[]  CS8Rot=[]  CS9Pos=[]  CS9Rot=[]  CS10Pos=[]  CS10Rot=[]  CS11Pos=[]  CS11Rot=[]  CS12Pos=[]  CS12Rot=[]  CS13Pos=[]  CS13Rot=[]  CS14Pos=[]  CS14Rot=[]  CS15Pos=[]  CS15Rot=[]  CS16Pos=[]  CS16Rot=[]  CS17Pos=[]  CS17Rot=[]  CS18Pos=[]  CS18Rot=[]  CS19Pos=[]  CS19Rot=[]  CS20Pos=[]  CS20Rot=[]
  摇臂 : mblibv1/Bodies/Body  LConnTagsString=CS1|CS3|CS4|CS5  RConnTagsString=CS2  UpdateFromCAD=off  DialogClass=MechanicalBodyBlock  Mass=1  MassUnits=kg  InertiaUnits=kg*m^2  Inertia=eye(3)  Shape=Cylinder  ShapeDims=[1 1]  ShapeUnits=m  ShapeUse=false  Density=1  DensityUnits=kg/m^3  DensityUse=false  GraphicsMode=MACHINE_DEFAULT  BodyColorSelMode=MACHINE_DEFAULT  BodyColor=[1 0 0]  AttachedToCS=CG  CG=Left$CG$[xc1 yc1 zc1]$WORLD$WORLD$mm$[0 0 0]$Euler X-Y-Z$deg$WORLD$false$none  WorkingFrames=Left$CS1$[x4 y4 z4]$World$World$mm$[0 0 0]$Euler X-Y-Z$deg$WORLD$true$none#Right$CS2$[x3 y3 z3]$World$World$mm$[0 0 0]$Euler X-Y-Z$deg$WORLD$true$none#Left$CS3$[x5 y5 z5]$World$World$mm$[0 0 0]$Euler X-Y-Z$deg$WORLD$true$none#Left$CS4$[x5 y5 z5]$World$World$mm$[0 0 0]$Euler X-Y-Z$deg$WORLD$true$none#Left$CS5$[x7 y7 z7]$World$World$mm$[0 0 0]$Euler X-Y-Z$deg$WORLD$true$none  CGPos=[xc1 yc1 zc1]  CGRot=[0 0 0]  CS0Pos=[]  CS0Rot=[]  CS1Pos=[x4 y4 z4]  CS1Rot=[0 0 0]  CS2Pos=[x3 y3 z3]  CS2Rot=[0 0 0]  CS3Pos=[x5 y5 z5]  CS3Rot=[0 0 0]  CS4Pos=[x5 y5 z5]  CS4Rot=[0 0 0]  CS5Pos=[x7 y7 z7]  CS5Rot=[0 0 0]  CS6Pos=[]  CS6Rot=[]  CS7Pos=[]  CS7Rot=[]  CS8Pos=[]  CS8Rot=[]  CS9Pos=[]  CS9Rot=[]  CS10Pos=[]  CS10Rot=[]  CS11Pos=[]  CS11Rot=[]  CS12Pos=[]  CS12Rot=[]  CS13Pos=[]  CS13Rot=[]  CS14Pos=[]  CS14Rot=[]  CS15Pos=[]  CS15Rot=[]  CS16Pos=[]  CS16Rot=[]  CS17Pos=[]  CS17Rot=[]  CS18Pos=[]  CS18Rot=[]  CS19Pos=[]  CS19Rot=[]  CS20Pos=[]  CS20Rot=[]
  摇臂车架接点 : mblibv1/Bodies/Ground  UpdateFromCAD=off  LeftPortType=env  RightPortType=workingframe  PhysicalDomain=Mechanical  DialogClass=GroundBlock  CoordPosition=[x4 y4 z4]  CoordPositionUnits=mm  StateVectorMgrId=-1  MachineId=[0 0]  ShowEnvPort=off  ParameterChecksum=[0 0 0 0]  TopologyChecksum=[0 0 0 0]
  摇臂阻尼接点 : mblibv1/Sensors &  Actuators/Body Sensor  UpdateFromCAD=off  PhysicalDomain=Mechanical  PortType=blob  Muxed=on  Pose=off  Angle=on  AngleUnits=deg  ArcVelocity=off  ArcVelocityUnits=deg/s  ArcAcceleration=off  ArcAccelerationUnits=deg/s^2  CoordPosition=on  CoordPositionUnits=mm  Velocity=off  VelocityUnits=mm/s  Acceleration=off  AccelerationUnits=m/s^2  Quaternion=on  QuaternionDT=off  QuaternionDDT=off  QuaternionUnits=off  OutputVector=[1]  ActiveIO=on  Width=3  DialogClass=MechanicalSensorBlock  ReferenceFrame=Absolute (World)
  Conn1 : PMIOPort  Port=1  Side=Right
  wires:
  摇臂阻尼接点/1 -> 5/1(In1)
  Joint Sensor3/1 -> To Workspace/1
  Joint Sensor/1 -> To Workspace1/1
  connections:
  推杆/RConn1 -- Spherical11/LConn1
  Spherical10/RConn1 -- Conn1/RConn1
  摇臂车架接点/RConn1 -- Revolute6/LConn1
  推杆/LConn1 -- Spherical10/LConn1
  摇臂/RConn1 -- Spherical11/RConn1
  Revolute6/RConn1 -- 摇臂/LConn1
  摇臂阻尼接点/LConn1 -- 摇臂/LConn3
  Body Spring & Damper/LConn1 -- Ground/RConn1
  Body Spring & Damper/RConn1 -- 摇臂/LConn2
  Joint Sensor3/LConn1 -- Revolute1/LConn2
  Revolute1/RConn1 -- 9‘/RConn1
  "l8 "/LConn1 -- Spherical1/RConn1
  Spherical2/RConn1 -- 摇臂/LConn4
  Spherical1/LConn1 -- l7/LConn1
  "l8 "/RConn1 -- Revolute1/LConn1
  Spherical2/LConn1 -- l7/RConn1
  Revolute6/LConn2 -- Joint Sensor/LConn1

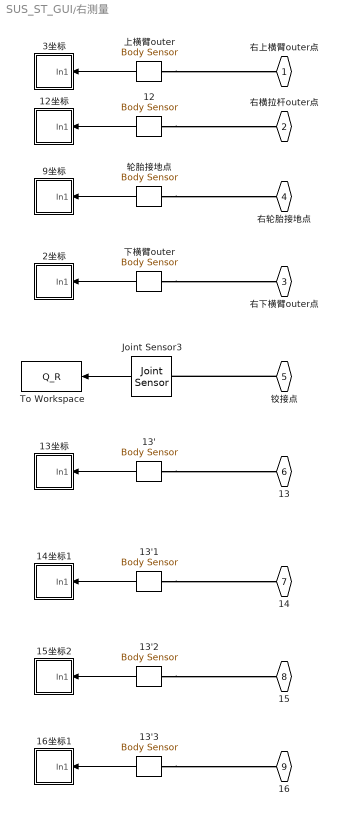
== system SUS_ST_GUI/右测量 ==
  " 12" : mblibv1/Sensors &  Actuators/Body Sensor  UpdateFromCAD=off  PhysicalDomain=Mechanical  PortType=blob  Muxed=on  Pose=off  Angle=on  AngleUnits=deg  ArcVelocity=off  ArcVelocityUnits=deg/s  ArcAcceleration=off  ArcAccelerationUnits=deg/s^2  CoordPosition=on  CoordPositionUnits=mm  Velocity=off  VelocityUnits=mm/s  Acceleration=off  AccelerationUnits=m/s^2  Quaternion=on  QuaternionDT=off  QuaternionDDT=off  QuaternionUnits=off  OutputVector=[1]  ActiveIO=on  Width=3  DialogClass=MechanicalSensorBlock  ReferenceFrame=Absolute (World)
  12坐标 : Subsystem
  13'{,1..3} (4 alike) : mblibv1/Sensors &  Actuators/Body Sensor  UpdateFromCAD=off  PhysicalDomain=Mechanical  PortType=blob  Muxed=on  Pose=off  Angle=on  AngleUnits=deg  ArcVelocity=off  ArcVelocityUnits=deg/s  ArcAcceleration=off  ArcAccelerationUnits=deg/s^2  CoordPosition=on  CoordPositionUnits=mm  Velocity=off  VelocityUnits=mm/s  Acceleration=off  AccelerationUnits=m/s^2  Quaternion=on  QuaternionDT=off  QuaternionDDT=off  QuaternionUnits=off  OutputVector=[1]  ActiveIO=on  Width=3  DialogClass=MechanicalSensorBlock  ReferenceFrame=Absolute (World)
  13坐标 : Subsystem
  14坐标1 : Subsystem
  15坐标2 : Subsystem
  16坐标1 : Subsystem
  2坐标 : Subsystem
  3坐标 : Subsystem
  9坐标 : Subsystem
  Joint Sensor3 : mblibv1/Sensors &  Actuators/Joint Sensor  RequirementInfo={} %GIDa_a4c87021_d943_4645_ab45_cd1622ee045f  UpdateFromCAD=off  PhysicalDomain=Mechanical  PortType=blob  Muxed=on  Pose=off  Angle=on  AngleUnits=deg  ArcVelocity=off  ArcVelocityUnits=deg/s  ArcAcceleration=off  ArcAccelerationUnits=deg/s^2  CoordPosition=on  CoordPositionUnits=m  Velocity=off  VelocityUnits=m/s  Acceleration=off  AccelerationUnits=m/s^2  Quaternion=on  QuaternionDT=off  QuaternionDDT=off  QuaternionUnits=off  OutputVector=[1]  ActiveIO=on  Width=4  DialogClass=MechanicalSensorBlock  Primitive=S  Force=off  ForceUnits=N  Torque=off  TorqueUnits=N*m  ReferenceFrame=Absolute (World)  ReactionSensedSide=Follower  ReactionReferenceFrame=Local (Body CS)  ReactionForce=off  ReactionForceUnits=N  ReactionMoment=off  ReactionMomentUnits=N*m
  To Workspace : ToWorkspace  VariableName=Q_R  SampleTime=-1
      settings: RequirementInfo={} %GIDa_adbb57f0_dee6_4cf8_9ce1_8989fbabbf75
  上横臂outer : mblibv1/Sensors &  Actuators/Body Sensor  UpdateFromCAD=off  PhysicalDomain=Mechanical  PortType=blob  Muxed=on  Pose=off  Angle=on  AngleUnits=deg  ArcVelocity=off  ArcVelocityUnits=deg/s  ArcAcceleration=off  ArcAccelerationUnits=deg/s^2  CoordPosition=on  CoordPositionUnits=mm  Velocity=off  VelocityUnits=mm/s  Acceleration=off  AccelerationUnits=m/s^2  Quaternion=on  QuaternionDT=off  QuaternionDDT=off  QuaternionUnits=off  OutputVector=[1]  ActiveIO=on  Width=3  DialogClass=MechanicalSensorBlock  ReferenceFrame=Absolute (World)
  下横臂outer : mblibv1/Sensors &  Actuators/Body Sensor  UpdateFromCAD=off  PhysicalDomain=Mechanical  PortType=blob  Muxed=on  Pose=off  Angle=on  AngleUnits=deg  ArcVelocity=off  ArcVelocityUnits=deg/s  ArcAcceleration=off  ArcAccelerationUnits=deg/s^2  CoordPosition=on  CoordPositionUnits=mm  Velocity=off  VelocityUnits=mm/s  Acceleration=off  AccelerationUnits=m/s^2  Quaternion=on  QuaternionDT=off  QuaternionDDT=off  QuaternionUnits=off  OutputVector=[1]  ActiveIO=on  Width=3  DialogClass=MechanicalSensorBlock  ReferenceFrame=Absolute (World)
  "轮胎接地点 " : mblibv1/Sensors &  Actuators/Body Sensor  UpdateFromCAD=off  PhysicalDomain=Mechanical  PortType=blob  Muxed=on  Pose=off  Angle=on  AngleUnits=deg  ArcVelocity=off  ArcVelocityUnits=deg/s  ArcAcceleration=off  ArcAccelerationUnits=deg/s^2  CoordPosition=on  CoordPositionUnits=mm  Velocity=off  VelocityUnits=mm/s  Acceleration=off  AccelerationUnits=m/s^2  Quaternion=on  QuaternionDT=off  QuaternionDDT=off  QuaternionUnits=off  OutputVector=[1]  ActiveIO=on  Width=3  DialogClass=MechanicalSensorBlock  ReferenceFrame=Absolute (World)
  右上横臂outer点 : PMIOPort  Port=1  Side=Right
  右横拉杆outer点 : PMIOPort  Port=2  Side=Right
  右下横臂outer点 : PMIOPort  Port=3  Side=Right
  右轮胎接地点 : PMIOPort  Port=4  Side=Right
  铰接点 : PMIOPort  Port=5  Side=Right
  13 : PMIOPort  Port=6  Side=Right
  14 : PMIOPort  Port=7  Side=Left
  15 : PMIOPort  Port=8  Side=Left
  16 : PMIOPort  Port=9  Side=Left
  wires:
  "轮胎接地点 "/1 -> 9坐标/1(In1)
  上横臂outer/1 -> 3坐标/1(In1)
  下横臂outer/1 -> 2坐标/1(In1)
  " 12"/1 -> 12坐标/1(In1)
  Joint Sensor3/1 -> To Workspace/1
  13'/1 -> 13坐标/1(In1)
  13'1/1 -> 14坐标1/1(In1)
  13'2/1 -> 15坐标2/1(In1)
  13'3/1 -> 16坐标1/1(In1)
  connections:
  "轮胎接地点 "/LConn1 -- 右轮胎接地点/RConn1
  上横臂outer/LConn1 -- 右上横臂outer点/RConn1
  下横臂outer/LConn1 -- 右下横臂outer点/RConn1
  " 12"/LConn1 -- 右横拉杆outer点/RConn1
  铰接点/RConn1 -- Joint Sensor3/LConn1
  13'/LConn1 -- 13/RConn1
  13'1/LConn1 -- 14/RConn1
  13'2/LConn1 -- 15/RConn1
  13'3/LConn1 -- 16/RConn1

== system SUS_ST_GUI/左上横臂 ==
  Revolute10 : mblibv1/Joints/Revolute  LConnTagsString=__newl0  RConnTagsString=__newr0  UpdateFromCAD=off  NumSAPorts=0  CutJoint=off  MarkAsCut=off  Primitives=prismatic  PrimitiveProps=R1$World$[cosd(T5) 0 sind(T5)]$revolute  DialogClass=JointBlock  R1Axis=[cosd(T5) 0 sind(T5)]
  Revolute7 : mblibv1/Joints/Revolute  LConnTagsString=__newl0  RConnTagsString=__newr0  UpdateFromCAD=off  NumSAPorts=0  CutJoint=off  MarkAsCut=off  Primitives=prismatic  PrimitiveProps=R1$World$[cosd(T5) 0 sind(T5)]$revolute  DialogClass=JointBlock  R1Axis=[cosd(T5) 0 sind(T5)]
  Spherical4 : mblibv1/Joints/Spherical  LConnTagsString=__newl0  RConnTagsString=__newr0  UpdateFromCAD=off  NumSAPorts=0  CutJoint=off  MarkAsCut=off  Primitives=spherical  PrimitiveProps=S$WORLD$[0 0 0]$spherical  DialogClass=JointBlock  SAxis=[0 0 0]
  上横臂1 : mblibv1/Bodies/Body  LConnTagsString=CS1|CS3  RConnTagsString=CS2  UpdateFromCAD=off  DialogClass=MechanicalBodyBlock  Mass=1  MassUnits=kg  InertiaUnits=kg*m^2  Inertia=eye(3)  Shape=Cylinder  ShapeDims=[1 1]  ShapeUnits=m  ShapeUse=false  Density=1  DensityUnits=kg/m^3  DensityUse=false  GraphicsMode=MACHINE_DEFAULT  BodyColorSelMode=MACHINE_DEFAULT  BodyColor=[1 0 0]  AttachedToCS=CG  CG=Left$CG$[XC3 -YC3 ZC3]$WORLD$WORLD$mm$[0 0 0]$Euler X-Y-Z$deg$WORLD$false$none  WorkingFrames=Left$CS1$[X5 -Y5 Z5]$World$World$mm$[0 0 0]$Euler X-Y-Z$deg$WORLD$true$none#Right$CS2$[X3 -Y3 Z3]$World$World$mm$[0 0 0]$Euler X-Y-Z$deg$WORLD$true$none#Left$CS3$[X6 -Y6 Z6]$World$World$mm$[0 0 0]$Euler X-Y-Z$deg$WORLD$true$none  CGPos=[XC3 -YC3 ZC3]  CGRot=[0 0 0]  CS0Pos=[]  CS0Rot=[]  CS1Pos=[X5 -Y5 Z5]  CS1Rot=[0 0 0]  CS2Pos=[X3 -Y3 Z3]  CS2Rot=[0 0 0]  CS3Pos=[X6 -Y6 Z6]  CS3Rot=[0 0 0]  CS4Pos=[]  CS4Rot=[]  CS5Pos=[]  CS5Rot=[]  CS6Pos=[]  CS6Rot=[]  CS7Pos=[]  CS7Rot=[]  CS8Pos=[]  CS8Rot=[]  CS9Pos=[]  CS9Rot=[]  CS10Pos=[]  CS10Rot=[]  CS11Pos=[]  CS11Rot=[]  CS12Pos=[]  CS12Rot=[]  CS13Pos=[]  CS13Rot=[]  CS14Pos=[]  CS14Rot=[]  CS15Pos=[]  CS15Rot=[]  CS16Pos=[]  CS16Rot=[]  CS17Pos=[]  CS17Rot=[]  CS18Pos=[]  CS18Rot=[]  CS19Pos=[]  CS19Rot=[]  CS20Pos=[]  CS20Rot=[]
  上横臂inner前点1 : mblibv1/Bodies/Ground  UpdateFromCAD=off  LeftPortType=env  RightPortType=workingframe  PhysicalDomain=Mechanical  DialogClass=GroundBlock  CoordPosition=[X5 -Y5 Z5]  CoordPositionUnits=mm  StateVectorMgrId=-1  MachineId=[0 0]  ShowEnvPort=off  ParameterChecksum=[0 0 0 0]  TopologyChecksum=[0 0 0 0]
  上横臂inner后点1 : mblibv1/Bodies/Ground  UpdateFromCAD=off  LeftPortType=env  RightPortType=workingframe  PhysicalDomain=Mechanical  DialogClass=GroundBlock  CoordPosition=[X6 -Y6 Z6]  CoordPositionUnits=mm  StateVectorMgrId=-1  MachineId=[0 0]  ShowEnvPort=off  ParameterChecksum=[0 0 0 0]  TopologyChecksum=[0 0 0 0]
  Conn1 : PMIOPort  Port=1  Side=Left
  connections:
  Revolute7/LConn1 -- 上横臂inner前点1/RConn1
  上横臂1/RConn1 -- Spherical4/LConn1
  上横臂inner后点1/RConn1 -- Revolute10/LConn1
  Spherical4/RConn1 -- Conn1/RConn1
  上横臂1/LConn1 -- Revolute7/RConn1
  上横臂1/LConn2 -- Revolute10/RConn1

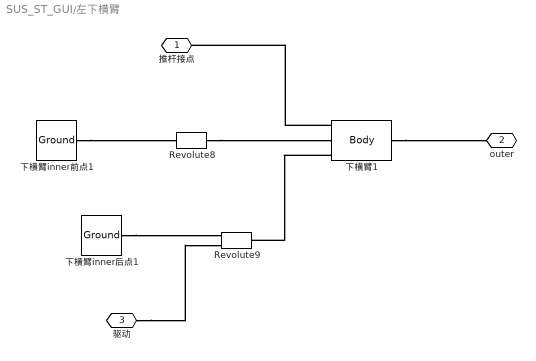
== system SUS_ST_GUI/左下横臂 ==
  Revolute8 : mblibv1/Joints/Revolute  LConnTagsString=__newl0  RConnTagsString=__newr0  UpdateFromCAD=off  NumSAPorts=0  CutJoint=off  MarkAsCut=off  Primitives=prismatic  PrimitiveProps=R1$World$[cosd(T6) 0 sind(T6)]$revolute  DialogClass=JointBlock  R1Axis=[cosd(T6) 0 sind(T6)]
  Revolute9 : mblibv1/Joints/Revolute  LConnTagsString=__newl0|SA1  RConnTagsString=__newr0  UpdateFromCAD=off  NumSAPorts=1  CutJoint=off  MarkAsCut=off  Primitives=prismatic  PrimitiveProps=R1$World$[cosd(T6) 0 sind(T6)]$revolute  DialogClass=JointBlock  R1Axis=[cosd(T6) 0 sind(T6)]
  下横臂1 : mblibv1/Bodies/Body  LConnTagsString=CS3|CS1|CS4  RConnTagsString=CS2  UpdateFromCAD=off  DialogClass=MechanicalBodyBlock  Mass=1  MassUnits=kg  InertiaUnits=kg*m^2  Inertia=eye(3)  Shape=Cylinder  ShapeDims=[1 1]  ShapeUnits=m  ShapeUse=false  Density=1  DensityUnits=kg/m^3  DensityUse=false  GraphicsMode=MACHINE_DEFAULT  BodyColorSelMode=MACHINE_DEFAULT  BodyColor=[1 0 0]  AttachedToCS=CG  CG=Left$CG$[XC1 -YC1 ZC1]$WORLD$WORLD$mm$[0 0 0]$Euler X-Y-Z$deg$WORLD$false$none  WorkingFrames=Left$CS3$[x2 -y2 z2]$WORLD$WORLD$mm$[0 0 0]$Euler X-Y-Z$deg$WORLD$true$none#Left$CS1$[X7 -Y7 Z7]$World$World$mm$[0 0 0]$Euler X-Y-Z$deg$WORLD$true$none#Right$CS2$[X2 -Y2 Z2]$World$World$mm$[-IN CA 0]$Euler X-Y-Z$deg$WORLD$true$none#Left$CS4$[X8 -Y8 Z8]$World$World$mm$[0 0 0]$Euler X-Y-Z$deg$WORLD$true$none  CGPos=[XC1 -YC1 ZC1]  CGRot=[0 0 0]  CS0Pos=[]  CS0Rot=[]  CS1Pos=[X7 -Y7 Z7]  CS1Rot=[0 0 0]  CS2Pos=[X2 -Y2 Z2]  CS2Rot=[-IN CA 0]  CS3Pos=[x2 -y2 z2]  CS3Rot=[0 0 0]  CS4Pos=[X8 -Y8 Z8]  CS4Rot=[0 0 0]  CS5Pos=[]  CS5Rot=[]  CS6Pos=[]  CS6Rot=[]  CS7Pos=[]  CS7Rot=[]  CS8Pos=[]  CS8Rot=[]  CS9Pos=[]  CS9Rot=[]  CS10Pos=[]  CS10Rot=[]  CS11Pos=[]  CS11Rot=[]  CS12Pos=[]  CS12Rot=[]  CS13Pos=[]  CS13Rot=[]  CS14Pos=[]  CS14Rot=[]  CS15Pos=[]  CS15Rot=[]  CS16Pos=[]  CS16Rot=[]  CS17Pos=[]  CS17Rot=[]  CS18Pos=[]  CS18Rot=[]  CS19Pos=[]  CS19Rot=[]  CS20Pos=[]  CS20Rot=[]
  下横臂inner前点1 : mblibv1/Bodies/Ground  UpdateFromCAD=off  LeftPortType=env  RightPortType=workingframe  PhysicalDomain=Mechanical  DialogClass=GroundBlock  CoordPosition=[X7 -Y7 Z7]  CoordPositionUnits=mm  StateVectorMgrId=-1  MachineId=[0 0]  ShowEnvPort=off  ParameterChecksum=[0 0 0 0]  TopologyChecksum=[0 0 0 0]
  下横臂inner后点1 : mblibv1/Bodies/Ground  UpdateFromCAD=off  LeftPortType=env  RightPortType=workingframe  PhysicalDomain=Mechanical  DialogClass=GroundBlock  CoordPosition=[X8 -Y8 Z8]  CoordPositionUnits=mm  StateVectorMgrId=-1  MachineId=[0 0]  ShowEnvPort=off  ParameterChecksum=[0 0 0 0]  TopologyChecksum=[0 0 0 0]
  推杆接点 : PMIOPort  Port=1  Side=Left
  outer : PMIOPort  Port=2  Side=Right
  驱动 : PMIOPort  Port=3  Side=Left
  connections:
  下横臂1/LConn1 -- 推杆接点/RConn1
  下横臂inner前点1/RConn1 -- Revolute8/LConn1
  下横臂1/LConn3 -- Revolute9/RConn1
  Revolute8/RConn1 -- 下横臂1/LConn2
  下横臂inner后点1/RConn1 -- Revolute9/LConn1
  下横臂1/RConn1 -- outer/RConn1
  驱动/RConn1 -- Revolute9/LConn2

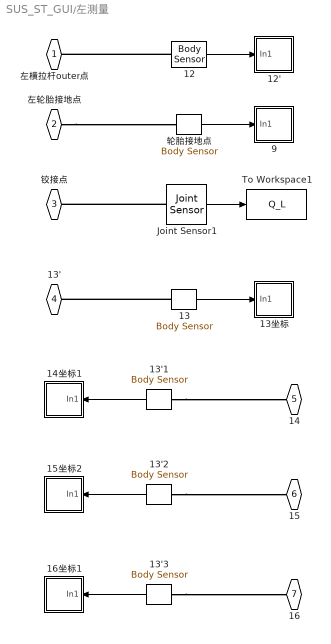
== system SUS_ST_GUI/左测量 ==
  12 : mblibv1/Sensors &  Actuators/Body Sensor  UpdateFromCAD=off  PhysicalDomain=Mechanical  PortType=blob  Muxed=on  Pose=off  Angle=on  AngleUnits=deg  ArcVelocity=off  ArcVelocityUnits=deg/s  ArcAcceleration=off  ArcAccelerationUnits=deg/s^2  CoordPosition=on  CoordPositionUnits=mm  Velocity=off  VelocityUnits=mm/s  Acceleration=off  AccelerationUnits=m/s^2  Quaternion=on  QuaternionDT=off  QuaternionDDT=off  QuaternionUnits=off  OutputVector=[1]  ActiveIO=on  Width=3  DialogClass=MechanicalSensorBlock  ReferenceFrame=Absolute (World)
  12' : Subsystem
  13 : mblibv1/Sensors &  Actuators/Body Sensor  UpdateFromCAD=off  PhysicalDomain=Mechanical  PortType=blob  Muxed=on  Pose=off  Angle=on  AngleUnits=deg  ArcVelocity=off  ArcVelocityUnits=deg/s  ArcAcceleration=off  ArcAccelerationUnits=deg/s^2  CoordPosition=on  CoordPositionUnits=mm  Velocity=off  VelocityUnits=mm/s  Acceleration=off  AccelerationUnits=m/s^2  Quaternion=on  QuaternionDT=off  QuaternionDDT=off  QuaternionUnits=off  OutputVector=[1]  ActiveIO=on  Width=3  DialogClass=MechanicalSensorBlock  ReferenceFrame=Absolute (World)
  13'1 : mblibv1/Sensors &  Actuators/Body Sensor  UpdateFromCAD=off  PhysicalDomain=Mechanical  PortType=blob  Muxed=on  Pose=off  Angle=on  AngleUnits=deg  ArcVelocity=off  ArcVelocityUnits=deg/s  ArcAcceleration=off  ArcAccelerationUnits=deg/s^2  CoordPosition=on  CoordPositionUnits=mm  Velocity=off  VelocityUnits=mm/s  Acceleration=off  AccelerationUnits=m/s^2  Quaternion=on  QuaternionDT=off  QuaternionDDT=off  QuaternionUnits=off  OutputVector=[1]  ActiveIO=on  Width=3  DialogClass=MechanicalSensorBlock  ReferenceFrame=Absolute (World)
  13'2 : mblibv1/Sensors &  Actuators/Body Sensor  UpdateFromCAD=off  PhysicalDomain=Mechanical  PortType=blob  Muxed=on  Pose=off  Angle=on  AngleUnits=deg  ArcVelocity=off  ArcVelocityUnits=deg/s  ArcAcceleration=off  ArcAccelerationUnits=deg/s^2  CoordPosition=on  CoordPositionUnits=mm  Velocity=off  VelocityUnits=mm/s  Acceleration=off  AccelerationUnits=m/s^2  Quaternion=on  QuaternionDT=off  QuaternionDDT=off  QuaternionUnits=off  OutputVector=[1]  ActiveIO=on  Width=3  DialogClass=MechanicalSensorBlock  ReferenceFrame=Absolute (World)
  13'3 : mblibv1/Sensors &  Actuators/Body Sensor  UpdateFromCAD=off  PhysicalDomain=Mechanical  PortType=blob  Muxed=on  Pose=off  Angle=on  AngleUnits=deg  ArcVelocity=off  ArcVelocityUnits=deg/s  ArcAcceleration=off  ArcAccelerationUnits=deg/s^2  CoordPosition=on  CoordPositionUnits=mm  Velocity=off  VelocityUnits=mm/s  Acceleration=off  AccelerationUnits=m/s^2  Quaternion=on  QuaternionDT=off  QuaternionDDT=off  QuaternionUnits=off  OutputVector=[1]  ActiveIO=on  Width=3  DialogClass=MechanicalSensorBlock  ReferenceFrame=Absolute (World)
  13坐标 : Subsystem
  14坐标1 : Subsystem
  15坐标2 : Subsystem
  16坐标1 : Subsystem
  9 : Subsystem
  Joint Sensor1 : mblibv1/Sensors &  Actuators/Joint Sensor  UpdateFromCAD=off  PhysicalDomain=Mechanical  PortType=blob  Muxed=on  Pose=off  Angle=on  AngleUnits=deg  ArcVelocity=off  ArcVelocityUnits=deg/s  ArcAcceleration=off  ArcAccelerationUnits=deg/s^2  CoordPosition=on  CoordPositionUnits=m  Velocity=off  VelocityUnits=m/s  Acceleration=off  AccelerationUnits=m/s^2  Quaternion=on  QuaternionDT=off  QuaternionDDT=off  QuaternionUnits=off  OutputVector=[1]  ActiveIO=on  Width=4  DialogClass=MechanicalSensorBlock  Primitive=S  Force=off  ForceUnits=N  Torque=off  TorqueUnits=N*m  ReferenceFrame=Absolute (World)  ReactionSensedSide=Base  ReactionReferenceFrame=Local (Body CS)  ReactionForce=off  ReactionForceUnits=N  ReactionMoment=off  ReactionMomentUnits=N*m
  To Workspace1 : ToWorkspace  VariableName=Q_L  SampleTime=-1
  "轮胎接地点 " : mblibv1/Sensors &  Actuators/Body Sensor  UpdateFromCAD=off  PhysicalDomain=Mechanical  PortType=blob  Muxed=on  Pose=off  Angle=on  AngleUnits=deg  ArcVelocity=off  ArcVelocityUnits=deg/s  ArcAcceleration=off  ArcAccelerationUnits=deg/s^2  CoordPosition=on  CoordPositionUnits=mm  Velocity=off  VelocityUnits=mm/s  Acceleration=off  AccelerationUnits=m/s^2  Quaternion=on  QuaternionDT=off  QuaternionDDT=off  QuaternionUnits=off  OutputVector=[1]  ActiveIO=on  Width=3  DialogClass=MechanicalSensorBlock  ReferenceFrame=Absolute (World)
  左横拉杆outer点 : PMIOPort  Port=1  Side=Left
  左轮胎接地点 : PMIOPort  Port=2  Side=Left
  铰接点 : PMIOPort  Port=3  Side=Left
  13' : PMIOPort  Port=4  Side=Left
  14 : PMIOPort  Port=5  Side=Right
  15 : PMIOPort  Port=6  Side=Right
  16 : PMIOPort  Port=7  Side=Right
  wires:
  Joint Sensor1/1 -> To Workspace1/1
  12/1 -> 12'/1(In1)
  "轮胎接地点 "/1 -> 9/1(In1)
  13/1 -> 13坐标/1(In1)
  13'1/1 -> 14坐标1/1(In1)
  13'2/1 -> 15坐标2/1(In1)
  13'3/1 -> 16坐标1/1(In1)
  connections:
  左轮胎接地点/RConn1 -- "轮胎接地点 "/LConn1
  Joint Sensor1/LConn1 -- 铰接点/RConn1
  12/LConn1 -- 左横拉杆outer点/RConn1
  13/LConn1 -- 13'/RConn1
  13'1/LConn1 -- 14/RConn1
  13'2/LConn1 -- 15/RConn1
  13'3/LConn1 -- 16/RConn1
